simulink model "CAN_basics"  (R2019a)
settings: Solver=FixedStepAuto  StartTime=0.0  StopTime=inf  RelTol=1e-3
InitFcn:
  | InitFcn
undefined symbols (not defined in the file or in its folder): CAN_ID_Frequencydata, CAN_ID_RAW_A0, CAN_ID_RAW_A1, CAN_ID_RAW_B0, CAN_ID_RAW_B1, CAN_ID_RAW_C0, CAN_ID_RAW_C1, CAN_ID_RAW_D0, CAN_ID_RAW_D1, CAN_ID_Timedata, canChannel
libraries: etargetslib x26, canmsglib x18, canlib x9, simulink x2
settings Model: Creator=abl  LastModifiedBy=abl

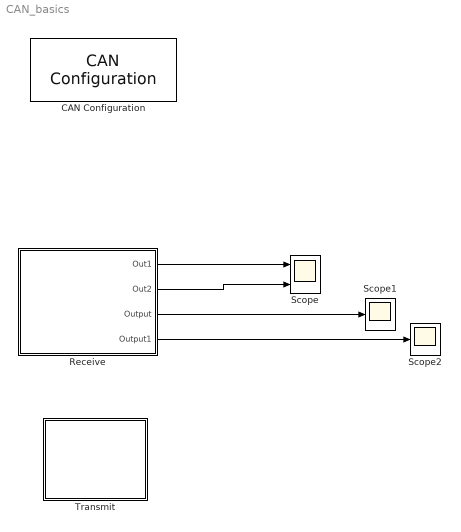
== system CAN_basics ==
  CAN Configuration : canlib/CAN Configuration  BlockHandle=2.0001  DeviceMenu=Vector VN1610 1 (Channel 1)  Device=Vector VN1610 1 (Channel 1)  ObjConstructor=canChannel('Vector', 'VN1610 1', 1)  BusSpeed=500000  EnableBitParameters=off  SJW=1  TSEG1=4  TSEG2=3  NSamples=1  AckMode=Normal
      settings: SourceProductName=Vehicle Network Toolbox  SourceProductBaseCode=VN
  Receive : Subsystem
  Scope : Scope  NumInputPorts=2
  Scope1 : Scope
  Scope2 : Scope
  Transmit : Subsystem
  wires:
  Receive/1(Out1) -> Scope/1
  Receive/2(Out2) -> Scope/2
  Receive/3(Output) -> Scope1/1
  Receive/4(Output1) -> Scope2/1

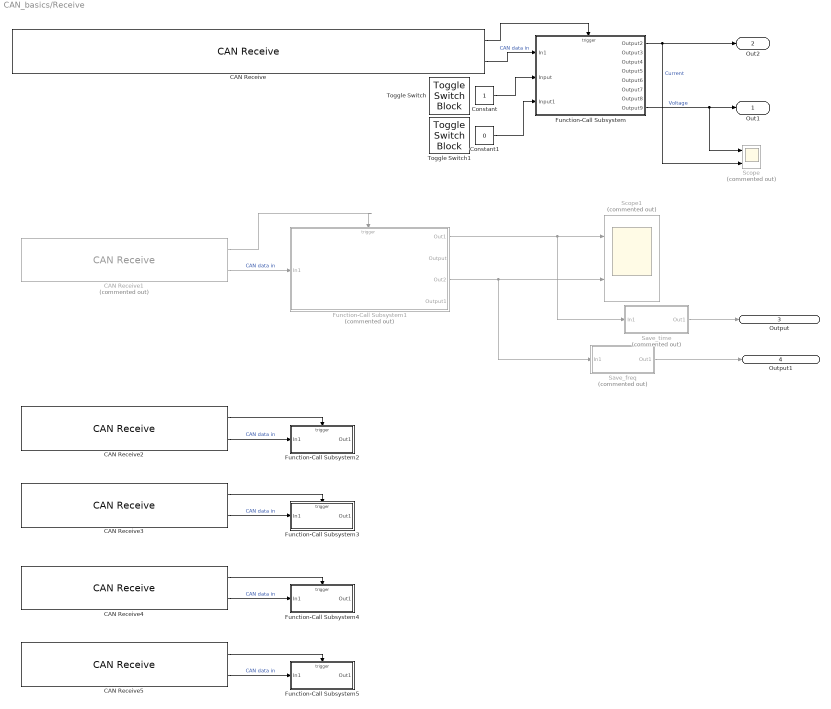
== system CAN_basics/Receive ==
  CAN Receive : canlib/CAN Receive  BlockHandle=4.0001  DeviceMenu=Vector VN1610 1 (Channel 1)  Device=Vector VN1610 1 (Channel 1)  ObjConstructor=canChannel('Vector', 'VN1610 1', 1)  EnableStandardIDsFilter=off  StandardIDs=[CAN_ID_RAW_A0;CAN_ID_RAW_A1;CAN_ID_RAW_B0;CAN_ID_RAW_B1;CAN_ID_RAW_C0;CAN_ID_RAW_C1;CAN_ID_RAW_D0;CAN_ID_RAW_D1]  EnableExtendedIDsFilter=off  ExtendedIDs=0  SampleTime=-1  MsgsPerTimestep=all  StdIDsCombo=Allow only  ExtIDsCombo=Block all  InternalFilterUpdateStatus=on  BusOutput=off
      settings: SourceProductName=Vehicle Network Toolbox  SourceProductBaseCode=VN
  CAN Receive1 : canlib/CAN Receive  Commented=on  BlockHandle=5.0001  DeviceMenu=Vector VN1610 1 (Channel 1)  Device=Vector VN1610 1 (Channel 1)  ObjConstructor=canChannel('Vector', 'VN1610 1', 1)  EnableStandardIDsFilter=off  StandardIDs=[CAN_ID_Timedata;CAN_ID_Frequencydata]  EnableExtendedIDsFilter=off  ExtendedIDs=0  SampleTime=-1  MsgsPerTimestep=all  StdIDsCombo=Allow only  ExtIDsCombo=Block all  InternalFilterUpdateStatus=on  BusOutput=off
      settings: SourceProductName=Vehicle Network Toolbox  SourceProductBaseCode=VN
  CAN Receive2 : canlib/CAN Receive  BlockHandle=6.0001  DeviceMenu=Vector VN1610 1 (Channel 1)  Device=Vector VN1610 1 (Channel 1)  ObjConstructor=canChannel('Vector', 'VN1610 1', 1)  EnableStandardIDsFilter=off  StandardIDs=CAN_ID_Timedata  EnableExtendedIDsFilter=off  ExtendedIDs=0  SampleTime=-1  MsgsPerTimestep=all  StdIDsCombo=Allow only  ExtIDsCombo=Block all  InternalFilterUpdateStatus=on  BusOutput=off
      settings: SourceProductName=Vehicle Network Toolbox  SourceProductBaseCode=VN
  CAN Receive3 : canlib/CAN Receive  BlockHandle=7.0001  DeviceMenu=Vector VN1610 1 (Channel 1)  Device=Vector VN1610 1 (Channel 1)  ObjConstructor=canChannel('Vector', 'VN1610 1', 1)  EnableStandardIDsFilter=off  StandardIDs=CAN_ID_Frequencydata  EnableExtendedIDsFilter=off  ExtendedIDs=0  SampleTime=-1  MsgsPerTimestep=all  StdIDsCombo=Allow only  ExtIDsCombo=Block all  InternalFilterUpdateStatus=on  BusOutput=off
      settings: SourceProductName=Vehicle Network Toolbox  SourceProductBaseCode=VN
  CAN Receive4 : canlib/CAN Receive  BlockHandle=1226.0002  DeviceMenu=Vector VN1610 1 (Channel 1)  Device=Vector VN1610 1 (Channel 1)  ObjConstructor=canChannel('Vector', 'VN1610 1', 1)  EnableStandardIDsFilter=off  StandardIDs=CAN_ID_Timedata_float  EnableExtendedIDsFilter=off  ExtendedIDs=0  SampleTime=-1  MsgsPerTimestep=1  StdIDsCombo=Allow only  ExtIDsCombo=Block all  InternalFilterUpdateStatus=on  BusOutput=off
      settings: SourceProductName=Vehicle Network Toolbox  SourceProductBaseCode=VN
  CAN Receive5 : canlib/CAN Receive  BlockHandle=1227.0002  DeviceMenu=Vector VN1610 1 (Channel 1)  Device=Vector VN1610 1 (Channel 1)  ObjConstructor=canChannel('Vector', 'VN1610 1', 1)  EnableStandardIDsFilter=off  StandardIDs=CAN_ID_Frequencydata_float  EnableExtendedIDsFilter=off  ExtendedIDs=0  SampleTime=-1  MsgsPerTimestep=1  StdIDsCombo=Allow only  ExtIDsCombo=Block all  InternalFilterUpdateStatus=on  BusOutput=off
      settings: SourceProductName=Vehicle Network Toolbox  SourceProductBaseCode=VN
  Constant : Constant
  Constant1 : Constant  Value=0
  Function-Call Subsystem : Subsystem  TreatAsAtomicUnit=on
  Function-Call Subsystem1 : Subsystem  Commented=on  TreatAsAtomicUnit=on
  Function-Call Subsystem2 : Subsystem  TreatAsAtomicUnit=on
  Function-Call Subsystem3 : Subsystem  TreatAsAtomicUnit=on
  Function-Call Subsystem4 : Subsystem  TreatAsAtomicUnit=on
  Function-Call Subsystem5 : Subsystem  TreatAsAtomicUnit=on
  Save_freq : Subsystem  Commented=on
  Save_time : Subsystem  Commented=on
  Scope : Scope  Commented=on  NumInputPorts=2
  Scope1 : Scope  Commented=on  NumInputPorts=2
  Toggle Switch : ToggleSwitchBlock  LabelPosition=Hide
      settings: Values={{'double', 'int16'}, [1 0]}
  Toggle Switch1 : ToggleSwitchBlock  LabelPosition=Hide
      settings: Values={{'8 CAN messages', '2 CAN messages'}, [1 0]}
  Out1 : Outport
  Out2 : Outport  Port=2
  Output : Outport  Port=3
  Output1 : Outport  Port=4
  wires:
  Function-Call Subsystem/8(Output9) -> Scope/1, Out1/1  "Voltage"
  Constant/1 -> Function-Call Subsystem/2(Input)
  CAN Receive/2 -> Function-Call Subsystem/1(In1)  "CAN data in"
  Constant1/1 -> Function-Call Subsystem/3(Input1)
  CAN Receive/1 -> Function-Call Subsystem/Trigger
  Function-Call Subsystem/1(Output2) -> Scope/2, Out2/1  "Current"
  CAN Receive1/1 -> Function-Call Subsystem1/Trigger
  CAN Receive1/2 -> Function-Call Subsystem1/1(In1)  "CAN data in"
  Function-Call Subsystem1/1(Out1) -> Save_time/1(In1), Scope1/1
  Function-Call Subsystem1/3(Out2) -> Save_freq/1(In1), Scope1/2
  Save_time/1(Out1) -> Output/1
  Save_freq/1(Out1) -> Output1/1
  CAN Receive2/2 -> Function-Call Subsystem2/1(In1)  "CAN data in"
  CAN Receive2/1 -> Function-Call Subsystem2/Trigger
  CAN Receive3/1 -> Function-Call Subsystem3/Trigger
  CAN Receive3/2 -> Function-Call Subsystem3/1(In1)  "CAN data in"
  CAN Receive4/1 -> Function-Call Subsystem4/Trigger
  CAN Receive4/2 -> Function-Call Subsystem4/1(In1)  "CAN data in"
  CAN Receive5/2 -> Function-Call Subsystem5/1(In1)  "CAN data in"
  CAN Receive5/1 -> Function-Call Subsystem5/Trigger

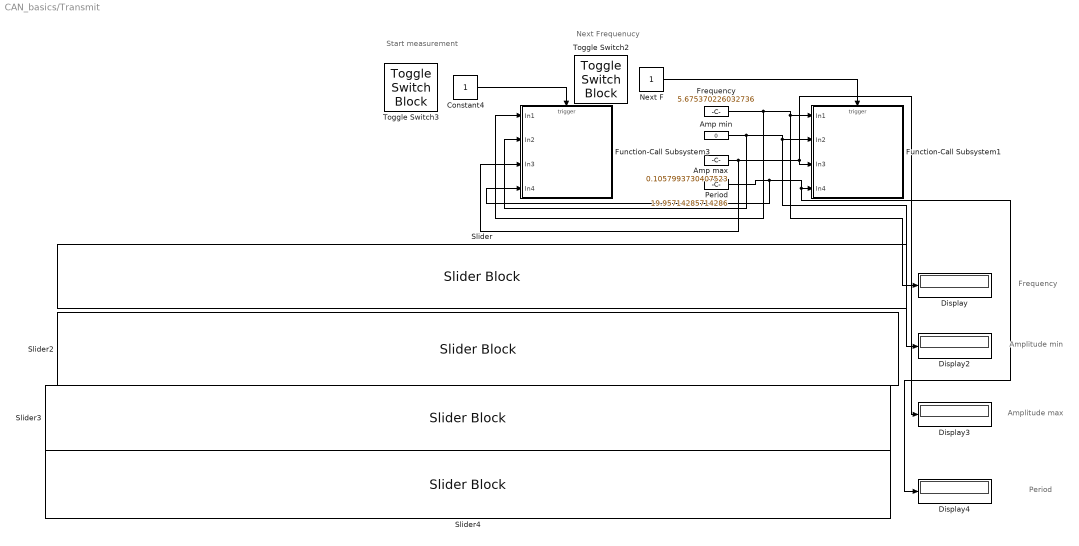
== system CAN_basics/Transmit ==
  note: Amplitude min
  note: Frequency
  note: Next Frequenucy
  note: Start measurement
  note: Amplitude max
  note: Period
  Amp max : Constant  Value=0.1057993730407523
  Amp min : Constant  Value=0
  Constant4 : Constant
  Display{,2..4} (4 alike) : Display
  Frequency : Constant  Value=5.675370226032736  OutDataTypeStr=uint16
  Function-Call Subsystem1 : Subsystem  TreatAsAtomicUnit=on
  Function-Call Subsystem3 : Subsystem  TreatAsAtomicUnit=on
  Next F : Constant
  Period : Constant  Value=19.95714285714286  OutDataTypeStr=uint16
  Slider : SliderBlock  ScaleMin=1  ScaleMax=4000
  Slider2 : SliderBlock  ScaleMax=5
  Slider3 : SliderBlock  ScaleMax=5
  Slider4 : SliderBlock  ScaleMin=1  ScaleMax=30  TickInterval=1
  Toggle Switch2 : ToggleSwitchBlock  LabelPosition=Hide
      settings: Values={{'Send message', 'Send message'}, [1 0]}
  Toggle Switch3 : ToggleSwitchBlock  LabelPosition=Hide
      settings: Values={{'Send message', 'Send message'}, [1 0]}
  wires:
  Amp min/1 -> Function-Call Subsystem3/2(In2), Display2/1, Function-Call Subsystem1/2(In2)
  Amp max/1 -> Display3/1, Function-Call Subsystem1/3(In3), Function-Call Subsystem3/3(In3)
  Period/1 -> Function-Call Subsystem3/4(In4), Display4/1, Function-Call Subsystem1/4(In4)
  Constant4/1 -> Function-Call Subsystem3/Trigger
  Next F/1 -> Function-Call Subsystem1/Trigger
  Frequency/1 -> Function-Call Subsystem3/1(In1), Display/1, Function-Call Subsystem1/1(In1)

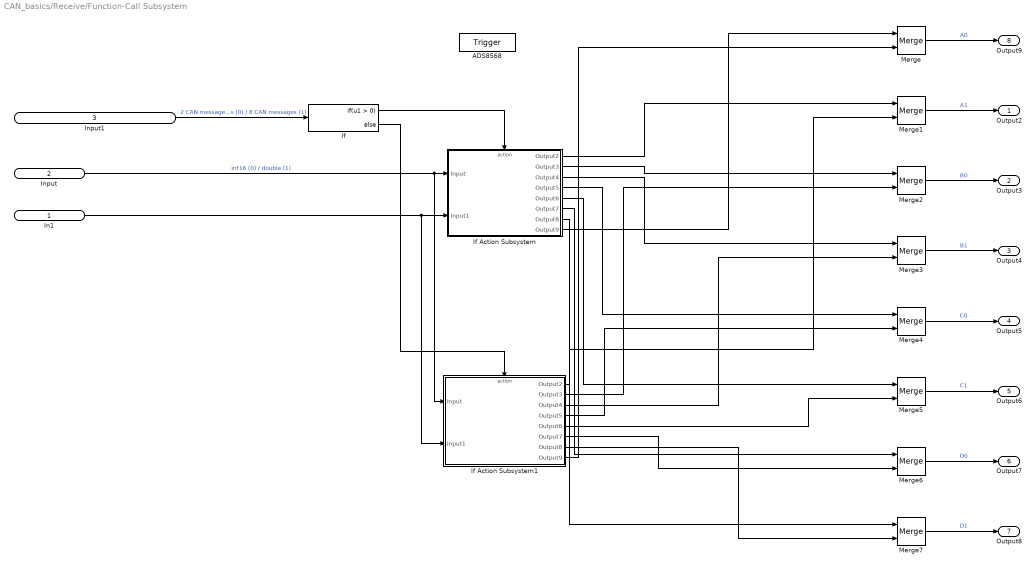
== system CAN_basics/Receive/Function-Call Subsystem ==
  In1 : Inport  Description=CAN data in
  Input : Inport  Port=2
  Input1 : Inport  Port=3
  ADS8568 : TriggerPort  TriggerType=function-call  VariantControl=Variant
  If : If
  If Action Subsystem : Subsystem  TreatAsAtomicUnit=on
  If Action Subsystem1 : Subsystem  TreatAsAtomicUnit=on
  Merge{,1..7} (8 alike) : Merge
  Output2 : Outport
  Output3 : Outport  Port=2
  Output4 : Outport  Port=3
  Output5 : Outport  Port=4
  Output6 : Outport  Port=5
  Output7 : Outport  Port=6
  Output8 : Outport  Port=7
  Output9 : Outport  Port=8
  wires:
  Input/1 -> If Action Subsystem1/1(Input), If Action Subsystem/1(Input)  "int16 (0) / double (1)"
  In1/1 -> If Action Subsystem1/2(Input1), If Action Subsystem/2(Input1)
  If/1 -> If Action Subsystem/Action
  Input1/1 -> If/1  "2 CAN messages (0) / 8 CAN messages (1)"
  If Action Subsystem/8(Output9) -> Merge/1
  If/2 -> If Action Subsystem1/Action
  Merge7/1 -> Output8/1  "D1"
  Merge6/1 -> Output7/1  "D0"
  Merge5/1 -> Output6/1  "C1"
  Merge4/1 -> Output5/1  "C0"
  Merge3/1 -> Output4/1  "B1"
  Merge2/1 -> Output3/1  "B0"
  Merge1/1 -> Output2/1  "A1"
  Merge/1 -> Output9/1  "A0"
  If Action Subsystem/1(Output2) -> Merge1/1
  If Action Subsystem/2(Output3) -> Merge2/1
  If Action Subsystem/3(Output4) -> Merge3/1
  If Action Subsystem/4(Output5) -> Merge4/1
  If Action Subsystem/5(Output6) -> Merge5/1
  If Action Subsystem/6(Output7) -> Merge6/1
  If Action Subsystem/7(Output8) -> Merge7/1
  If Action Subsystem1/8(Output9) -> Merge/2
  If Action Subsystem1/1(Output2) -> Merge1/2
  If Action Subsystem1/2(Output3) -> Merge2/2
  If Action Subsystem1/3(Output4) -> Merge3/2
  If Action Subsystem1/7(Output8) -> Merge7/2
  If Action Subsystem1/6(Output7) -> Merge6/2
  If Action Subsystem1/5(Output6) -> Merge5/2
  If Action Subsystem1/4(Output5) -> Merge4/2

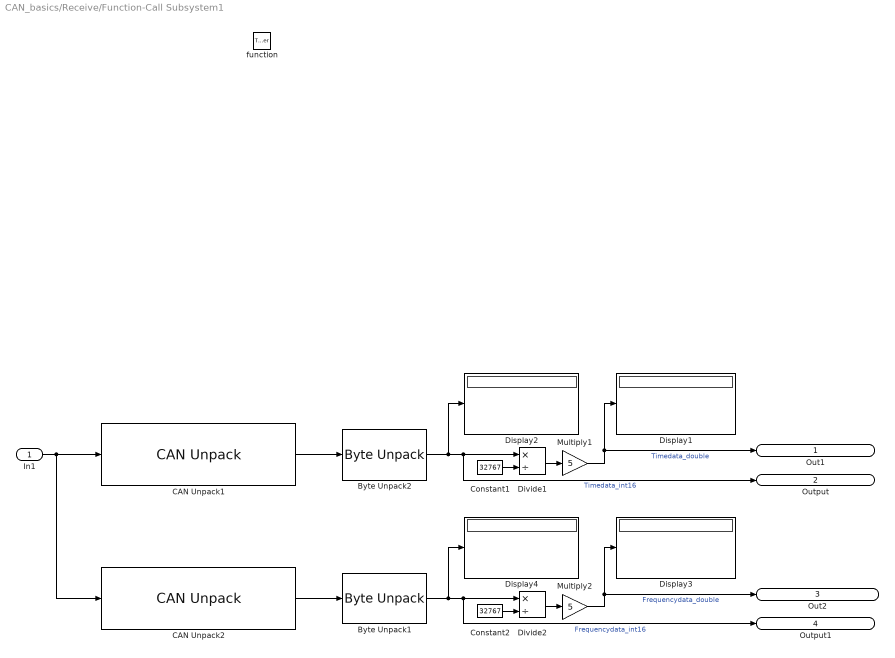
== system CAN_basics/Receive/Function-Call Subsystem1 ==
  In1 : Inport
  function : TriggerPort  TriggerType=function-call  VariantControl=Variant
  Byte Unpack1 : etargetslib/Byte Unpack  dimensions={[4]}  datatypes={'uint16'}  byteAlign=1
      settings: SourceProductName=MATLAB Coder
  Byte Unpack2 : etargetslib/Byte Unpack  dimensions={[4]}  datatypes={'uint16'}  byteAlign=1
      settings: SourceProductName=MATLAB Coder
  CAN Unpack1 : canmsglib/CAN Unpack  MsgList=(none)  MsgName=Timedata  MsgIDType=Standard (11-bit identifier)  MsgIdentifier=CAN_ID_Timedata  MsgLength=8  SignalInfo=A0$0$16$1$1$1$0$1$0$-Inf$Inf$#  NSignals=1  IDPort=off  TimestampPort=off  ErrorPort=off  RemotePort=off  LengthPort=off  StatusPort=off  StartBits=str2num('[int32(0)]')  SignalSizes=str2num('[int32(16)]')  ByteOrders=str2num('[int32(1)]')  DataTypes=str2num('[int32(1)]')  MultiplexTypes=str2num('[int32(1)]')  MultiplexValues=str2num('[double(0)]')  Factors=str2num('[double(1)]')  Offsets=str2num('[double(0)]')  Minimums=str2num('[double(-Inf)]')  Maximums=str2num('[double(Inf)]')  ApplyMinMax=off
      settings: SourceProductName=Vehicle Network Toolbox  SourceProductBaseCode=VN  DataFormat=raw data
  CAN Unpack2 : canmsglib/CAN Unpack  MsgList=(none)  MsgName=Frequencydata  MsgIDType=Standard (11-bit identifier)  MsgIdentifier=CAN_ID_Frequencydata  MsgLength=8  SignalInfo=A0$0$16$1$1$1$0$1$0$-Inf$Inf$#  NSignals=1  IDPort=off  TimestampPort=off  ErrorPort=off  RemotePort=off  LengthPort=off  StatusPort=off  StartBits=str2num('[int32(0)]')  SignalSizes=str2num('[int32(16)]')  ByteOrders=str2num('[int32(1)]')  DataTypes=str2num('[int32(1)]')  MultiplexTypes=str2num('[int32(1)]')  MultiplexValues=str2num('[double(0)]')  Factors=str2num('[double(1)]')  Offsets=str2num('[double(0)]')  Minimums=str2num('[double(-Inf)]')  Maximums=str2num('[double(Inf)]')  ApplyMinMax=off
      settings: SourceProductName=Vehicle Network Toolbox  SourceProductBaseCode=VN  DataFormat=raw data
  Constant1 : Constant  Value=32767
  Constant2 : Constant  Value=32767
  Display{1..4} (4 alike) : Display
      settings: Format=decimal (Stored Integer)
  Divide1 : Product  Inputs=*/
  Divide2 : Product  Inputs=*/
  Multiply1 : Gain  Gain=5
  Multiply2 : Gain  Gain=5
  Out1 : Outport
  Output : Outport  Port=2
  Out2 : Outport  Port=3
  Output1 : Outport  Port=4
  wires:
  CAN Unpack1/1 -> Byte Unpack2/1
  Divide1/1 -> Multiply1/1
  Multiply1/1 -> Out1/1, Display1/1  "Timedata_double"
  Constant1/1 -> Divide1/2
  Byte Unpack2/1 -> Output/1, Divide1/1, Display2/1  "Timedata_int16"
  Byte Unpack1/1 -> Output1/1, Divide2/1, Display4/1  "Frequencydata_int16"
  Constant2/1 -> Divide2/2
  Divide2/1 -> Multiply2/1
  Multiply2/1 -> Out2/1, Display3/1  "Frequencydata_double"
  CAN Unpack2/1 -> Byte Unpack1/1
  In1/1 -> CAN Unpack2/1, CAN Unpack1/1

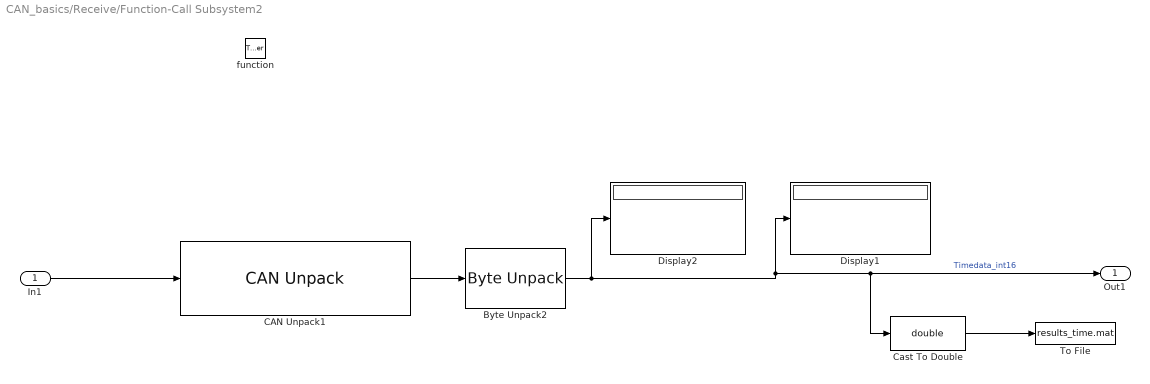
== system CAN_basics/Receive/Function-Call Subsystem2 ==
  In1 : Inport
  function : TriggerPort  TriggerType=function-call  VariantControl=Variant
  Byte Unpack2 : etargetslib/Byte Unpack  dimensions={[4]}  datatypes={'int16'}  byteAlign=1
      settings: SourceProductName=MATLAB Coder
  CAN Unpack1 : canmsglib/CAN Unpack  MsgList=(none)  MsgName=Timedata  MsgIDType=Standard (11-bit identifier)  MsgIdentifier=CAN_ID_Timedata  MsgLength=8  SignalInfo=A0$0$16$1$1$1$0$1$0$-Inf$Inf$#  NSignals=1  IDPort=off  TimestampPort=off  ErrorPort=off  RemotePort=off  LengthPort=off  StatusPort=off  StartBits=str2num('[int32(0)]')  SignalSizes=str2num('[int32(16)]')  ByteOrders=str2num('[int32(1)]')  DataTypes=str2num('[int32(1)]')  MultiplexTypes=str2num('[int32(1)]')  MultiplexValues=str2num('[double(0)]')  Factors=str2num('[double(1)]')  Offsets=str2num('[double(0)]')  Minimums=str2num('[double(-Inf)]')  Maximums=str2num('[double(Inf)]')  ApplyMinMax=off
      settings: SourceProductName=Vehicle Network Toolbox  SourceProductBaseCode=VN  DataFormat=raw data
  Cast To Double : DataTypeConversion  OutDataTypeStr=double
  Display1 : Display
      settings: Format=decimal (Stored Integer)
  Display2 : Display
      settings: Format=decimal (Stored Integer)
  To File : ToFile  Filename=results_time.mat  MatrixName=results_time
  Out1 : Outport
  wires:
  Byte Unpack2/1 -> Cast To Double/1, Out1/1, Display1/1, Display2/1  "Timedata_int16"
  CAN Unpack1/1 -> Byte Unpack2/1
  In1/1 -> CAN Unpack1/1
  Cast To Double/1 -> To File/1

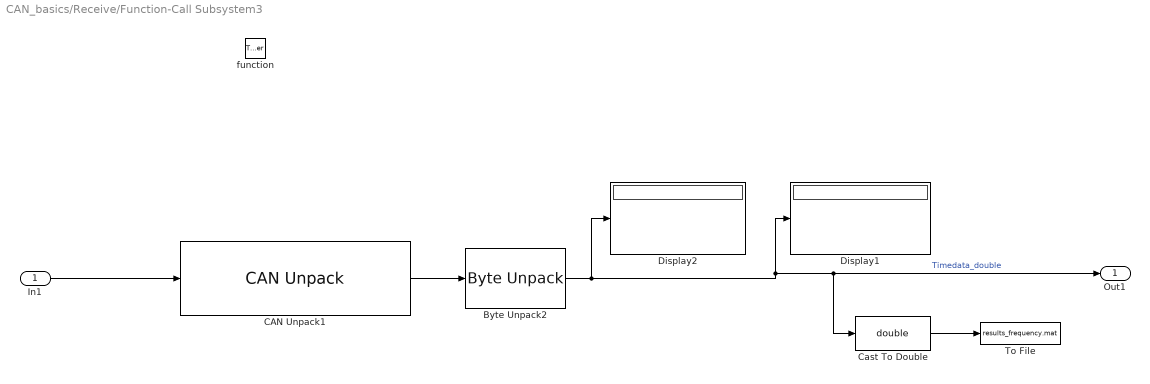
== system CAN_basics/Receive/Function-Call Subsystem3 ==
  In1 : Inport
  function : TriggerPort  TriggerType=function-call  VariantControl=Variant
  Byte Unpack2 : etargetslib/Byte Unpack  dimensions={[4]}  datatypes={'int16'}  byteAlign=1
      settings: SourceProductName=MATLAB Coder
  CAN Unpack1 : canmsglib/CAN Unpack  MsgList=(none)  MsgName=Frequencydata  MsgIDType=Standard (11-bit identifier)  MsgIdentifier=CAN_ID_Frequencydata  MsgLength=8  SignalInfo=A0$0$16$1$1$1$0$1$0$-Inf$Inf$#  NSignals=1  IDPort=off  TimestampPort=off  ErrorPort=off  RemotePort=off  LengthPort=off  StatusPort=off  StartBits=str2num('[int32(0)]')  SignalSizes=str2num('[int32(16)]')  ByteOrders=str2num('[int32(1)]')  DataTypes=str2num('[int32(1)]')  MultiplexTypes=str2num('[int32(1)]')  MultiplexValues=str2num('[double(0)]')  Factors=str2num('[double(1)]')  Offsets=str2num('[double(0)]')  Minimums=str2num('[double(-Inf)]')  Maximums=str2num('[double(Inf)]')  ApplyMinMax=off
      settings: SourceProductName=Vehicle Network Toolbox  SourceProductBaseCode=VN  DataFormat=raw data
  Cast To Double : DataTypeConversion  OutDataTypeStr=double
  Display1 : Display
      settings: Format=decimal (Stored Integer)
  Display2 : Display
      settings: Format=decimal (Stored Integer)
  To File : ToFile  Filename=results_frequency.mat  MatrixName=results_frequency
  Out1 : Outport
  wires:
  Byte Unpack2/1 -> Cast To Double/1, Out1/1, Display1/1, Display2/1  "Timedata_double"
  CAN Unpack1/1 -> Byte Unpack2/1
  In1/1 -> CAN Unpack1/1
  Cast To Double/1 -> To File/1

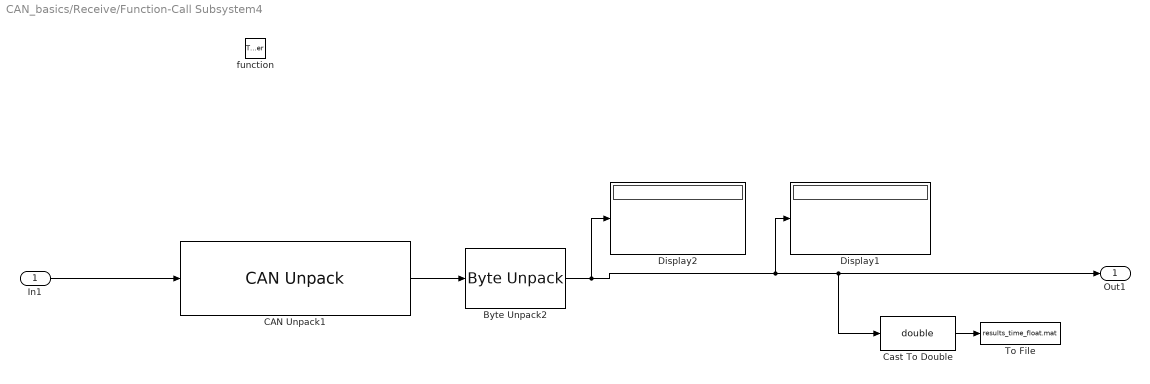
== system CAN_basics/Receive/Function-Call Subsystem4 ==
  In1 : Inport
  function : TriggerPort  TriggerType=function-call  VariantControl=Variant
  Byte Unpack2 : etargetslib/Byte Unpack  dimensions={[2]}  datatypes={'single'}  byteAlign=1
      settings: SourceProductName=MATLAB Coder
  CAN Unpack1 : canmsglib/CAN Unpack  MsgList=(none)  MsgName=Timedata  MsgIDType=Standard (11-bit identifier)  MsgIdentifier=CAN_ID_Timedata_float  MsgLength=8  SignalInfo=A0$0$16$1$1$1$0$1$0$-Inf$Inf$#  NSignals=1  IDPort=off  TimestampPort=off  ErrorPort=off  RemotePort=off  LengthPort=off  StatusPort=off  StartBits=str2num('[int32(0)]')  SignalSizes=str2num('[int32(16)]')  ByteOrders=str2num('[int32(1)]')  DataTypes=str2num('[int32(1)]')  MultiplexTypes=str2num('[int32(1)]')  MultiplexValues=str2num('[double(0)]')  Factors=str2num('[double(1)]')  Offsets=str2num('[double(0)]')  Minimums=str2num('[double(-Inf)]')  Maximums=str2num('[double(Inf)]')  ApplyMinMax=off
      settings: SourceProductName=Vehicle Network Toolbox  SourceProductBaseCode=VN  DataFormat=raw data
  Cast To Double : DataTypeConversion  OutDataTypeStr=double
  Display1 : Display
      settings: Format=decimal (Stored Integer)
  Display2 : Display
      settings: Format=decimal (Stored Integer)
  To File : ToFile  Filename=results_time_float.mat  MatrixName=results_time_float
  Out1 : Outport
  wires:
  Byte Unpack2/1 -> Cast To Double/1, Out1/1, Display1/1, Display2/1
  CAN Unpack1/1 -> Byte Unpack2/1
  In1/1 -> CAN Unpack1/1
  Cast To Double/1 -> To File/1

== system CAN_basics/Receive/Function-Call Subsystem5 ==
  In1 : Inport
  function : TriggerPort  TriggerType=function-call  VariantControl=Variant
  Byte Unpack2 : etargetslib/Byte Unpack  dimensions={[2]}  datatypes={'single'}  byteAlign=1
      settings: SourceProductName=MATLAB Coder
  CAN Unpack1 : canmsglib/CAN Unpack  MsgList=(none)  MsgName=Frequencydata  MsgIDType=Standard (11-bit identifier)  MsgIdentifier=CAN_ID_Frequencydata_float  MsgLength=8  SignalInfo=A0$0$16$1$1$1$0$1$0$-Inf$Inf$#  NSignals=1  IDPort=off  TimestampPort=off  ErrorPort=off  RemotePort=off  LengthPort=off  StatusPort=off  StartBits=str2num('[int32(0)]')  SignalSizes=str2num('[int32(16)]')  ByteOrders=str2num('[int32(1)]')  DataTypes=str2num('[int32(1)]')  MultiplexTypes=str2num('[int32(1)]')  MultiplexValues=str2num('[double(0)]')  Factors=str2num('[double(1)]')  Offsets=str2num('[double(0)]')  Minimums=str2num('[double(-Inf)]')  Maximums=str2num('[double(Inf)]')  ApplyMinMax=off
      settings: SourceProductName=Vehicle Network Toolbox  SourceProductBaseCode=VN  DataFormat=raw data
  Cast To Double : DataTypeConversion  OutDataTypeStr=double
  Display1 : Display
      settings: Format=decimal (Stored Integer)
  Display2 : Display
      settings: Format=decimal (Stored Integer)
  To File : ToFile  Filename=results_frequency_float.mat  MatrixName=results_frequency_float
  Out1 : Outport
  wires:
  Byte Unpack2/1 -> Display1/1, Out1/1, Cast To Double/1, Display2/1
  CAN Unpack1/1 -> Byte Unpack2/1
  In1/1 -> CAN Unpack1/1
  Cast To Double/1 -> To File/1

== system CAN_basics/Receive/Save_freq ==
  In1 : Inport
  Detect Change : simulink/Logic and Bit Operations/Detect Change  vinit=0  OutDataTypeStr=boolean
  Triggered Subsystem : Subsystem  TreatAsAtomicUnit=on
  Out1 : Outport
  wires:
  In1/1 -> Triggered Subsystem/1(In1), Detect Change/1
  Detect Change/1 -> Triggered Subsystem/Trigger
  Triggered Subsystem/1(Out1) -> Out1/1

== system CAN_basics/Receive/Save_time ==
  In1 : Inport
  Detect Change : simulink/Logic and Bit Operations/Detect Change  vinit=0  OutDataTypeStr=boolean
  Triggered Subsystem : Subsystem  TreatAsAtomicUnit=on
  Out1 : Outport
  wires:
  In1/1 -> Triggered Subsystem/1(In1), Detect Change/1
  Detect Change/1 -> Triggered Subsystem/Trigger
  Triggered Subsystem/1(Out1) -> Out1/1

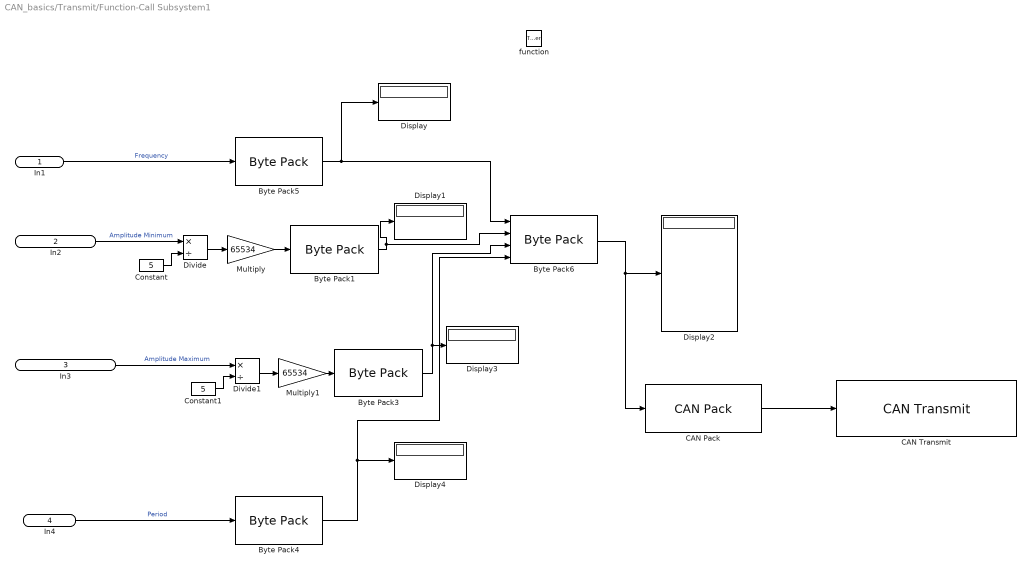
== system CAN_basics/Transmit/Function-Call Subsystem1 ==
  In1 : Inport
  In2 : Inport  Port=2
  In3 : Inport  Port=3
  In4 : Inport  Port=4
  function : TriggerPort  TriggerType=either  VariantControl=Variant
  Byte Pack{1,3..5} (4 alike) : etargetslib/Byte Pack  datatypes={'uint16'}  byteAlign=1
      settings: SourceProductName=MATLAB Coder
  Byte Pack6 : etargetslib/Byte Pack  datatypes={'uint8','uint8','uint8','uint8'}  byteAlign=1
      settings: SourceProductName=MATLAB Coder
  CAN Pack : canmsglib/CAN Pack  MsgList=(none)  MsgName=CAN Msg  MsgIDType=Standard (11-bit identifier)  MsgIdentifier=CAN_ID_Next_F  MsgLength=8  NSignals=0  StartBits=0  SignalSizes=0  ByteOrders=0  DataTypes=0  MultiplexTypes=0  MultiplexValues=0  Factors=0  Offsets=0  Minimums=0  Maximums=0  Remote=off  ApplyMinMax=off  BusOutput=off
      settings: SourceProductName=Vehicle Network Toolbox  SourceProductBaseCode=VN  DataFormat=raw data
  CAN Transmit : canlib/CAN Transmit  BlockHandle=541.0004  DeviceMenu=Vector VN1610 1 (Channel 1)  Device=Vector VN1610 1 (Channel 1)  ObjConstructor=canChannel('Vector', 'VN1610 1', 1)  EnablePeriodicTransmit=off  MessagePeriod=1.000
      settings: SourceProductName=Vehicle Network Toolbox  SourceProductBaseCode=VN
  Constant : Constant  Value=5
  Constant1 : Constant  Value=5
  Display{,1..4} (5 alike) : Display
  Divide : Product  Inputs=*/
  Divide1 : Product  Inputs=*/
  Multiply : Gain  Gain=65534  OutDataTypeStr=uint16
  Multiply1 : Gain  Gain=65534  OutDataTypeStr=uint16
  wires:
  CAN Pack/1 -> CAN Transmit/1
  In1/1 -> Byte Pack5/1  "Frequency"
  Byte Pack5/1 -> Byte Pack6/1, Display/1
  In2/1 -> Divide/1  "Amplitude Minimum"
  Constant/1 -> Divide/2
  Divide/1 -> Multiply/1
  Multiply/1 -> Byte Pack1/1
  Byte Pack1/1 -> Display1/1, Byte Pack6/2
  Byte Pack6/1 -> CAN Pack/1, Display2/1
  Divide1/1 -> Multiply1/1
  Constant1/1 -> Divide1/2
  In3/1 -> Divide1/1  "Amplitude Maximum"
  Multiply1/1 -> Byte Pack3/1
  Byte Pack3/1 -> Byte Pack6/3, Display3/1
  In4/1 -> Byte Pack4/1  "Period"
  Byte Pack4/1 -> Byte Pack6/4, Display4/1

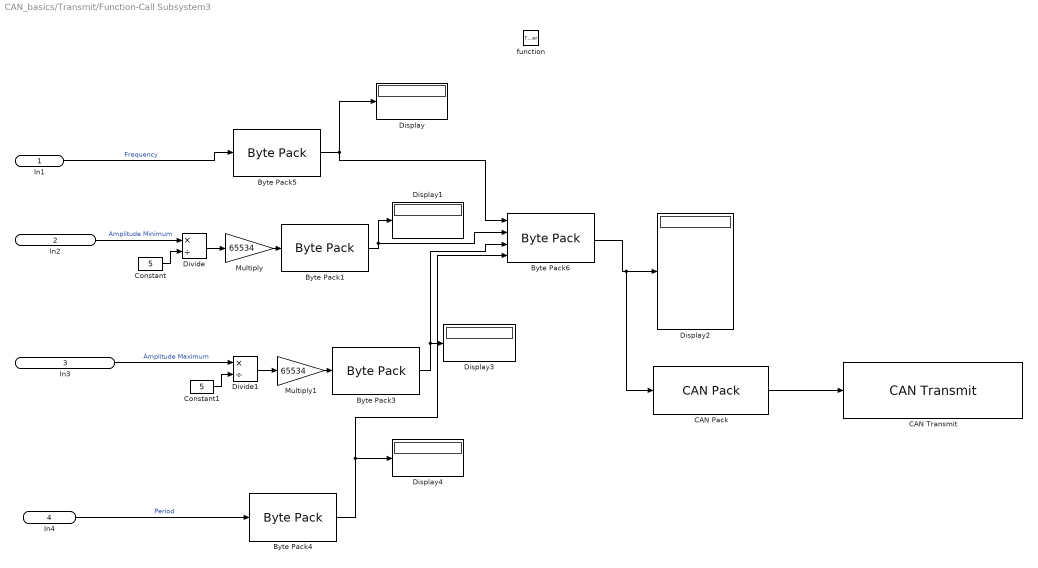
== system CAN_basics/Transmit/Function-Call Subsystem3 ==
  In1 : Inport
  In2 : Inport  Port=2
  In3 : Inport  Port=3
  In4 : Inport  Port=4
  function : TriggerPort  TriggerType=either  VariantControl=Variant
  Byte Pack{1,3..5} (4 alike) : etargetslib/Byte Pack  datatypes={'uint16'}  byteAlign=1
      settings: SourceProductName=MATLAB Coder
  Byte Pack6 : etargetslib/Byte Pack  datatypes={'uint8','uint8','uint8','uint8'}  byteAlign=2
      settings: SourceProductName=MATLAB Coder
  CAN Pack : canmsglib/CAN Pack  MsgList=(none)  MsgName=CAN Msg  MsgIDType=Standard (11-bit identifier)  MsgIdentifier=CAN_ID_Start_M  MsgLength=8  NSignals=0  StartBits=0  SignalSizes=0  ByteOrders=0  DataTypes=0  MultiplexTypes=0  MultiplexValues=0  Factors=0  Offsets=0  Minimums=0  Maximums=0  Remote=off  ApplyMinMax=off  BusOutput=off
      settings: SourceProductName=Vehicle Network Toolbox  SourceProductBaseCode=VN  DataFormat=raw data
  CAN Transmit : canlib/CAN Transmit  BlockHandle=591.0004  DeviceMenu=Vector VN1610 1 (Channel 1)  Device=Vector VN1610 1 (Channel 1)  ObjConstructor=canChannel('Vector', 'VN1610 1', 1)  EnablePeriodicTransmit=off  MessagePeriod=1.000
      settings: SourceProductName=Vehicle Network Toolbox  SourceProductBaseCode=VN
  Constant : Constant  Value=5
  Constant1 : Constant  Value=5
  Display{,1..4} (5 alike) : Display
  Divide : Product  Inputs=*/
  Divide1 : Product  Inputs=*/
  Multiply : Gain  Gain=65534  OutDataTypeStr=uint16
  Multiply1 : Gain  Gain=65534  OutDataTypeStr=uint16
  wires:
  CAN Pack/1 -> CAN Transmit/1
  In1/1 -> Byte Pack5/1  "Frequency"
  Byte Pack5/1 -> Byte Pack6/1, Display/1
  In2/1 -> Divide/1  "Amplitude Minimum"
  Constant/1 -> Divide/2
  Divide/1 -> Multiply/1
  Multiply/1 -> Byte Pack1/1
  Byte Pack1/1 -> Display1/1, Byte Pack6/2
  Byte Pack6/1 -> CAN Pack/1, Display2/1
  Divide1/1 -> Multiply1/1
  Constant1/1 -> Divide1/2
  In3/1 -> Divide1/1  "Amplitude Maximum"
  Multiply1/1 -> Byte Pack3/1
  Byte Pack3/1 -> Byte Pack6/3, Display3/1
  In4/1 -> Byte Pack4/1  "Period"
  Byte Pack4/1 -> Byte Pack6/4, Display4/1

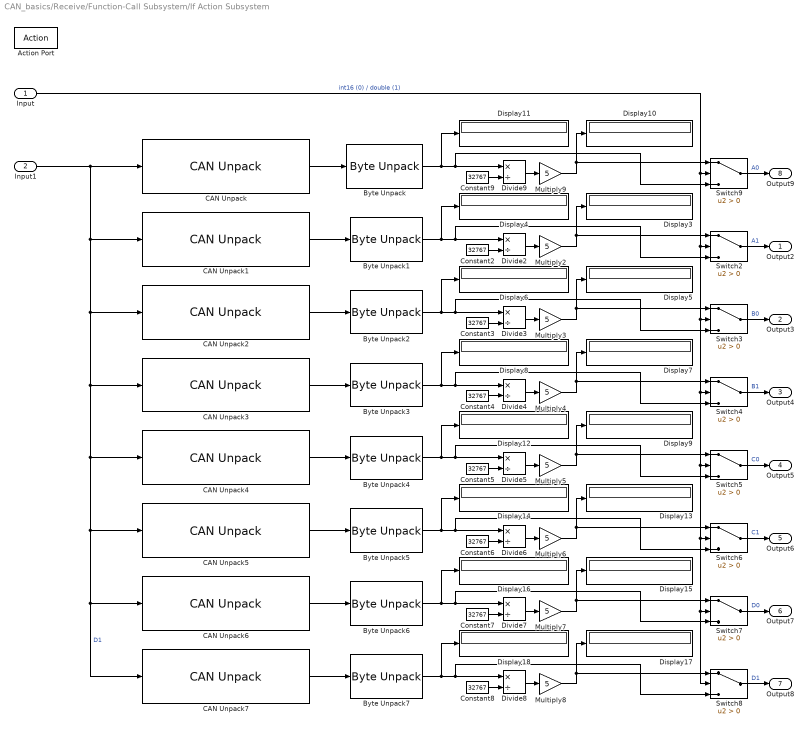
== system CAN_basics/Receive/Function-Call Subsystem/If Action Subsystem ==
  Input : Inport
  Input1 : Inport  Port=2
  Action Port : ActionPort  ActionPortLabel=if(u1 > 0)
  Byte Unpack{,1..7} (8 alike) : etargetslib/Byte Unpack  dimensions={[1]}  datatypes={'uint16'}  byteAlign=1
      settings: SourceProductName=MATLAB Coder
  CAN Unpack : canmsglib/CAN Unpack  MsgList=(none)  MsgName=ADC A0  MsgIDType=Standard (11-bit identifier)  MsgIdentifier=CAN_ID_RAW_A0  MsgLength=2  SignalInfo=A0$0$16$1$1$1$0$1$0$-Inf$Inf$#  NSignals=1  IDPort=off  TimestampPort=off  ErrorPort=off  RemotePort=off  LengthPort=off  StatusPort=off  StartBits=str2num('[int32(0)]')  SignalSizes=str2num('[int32(16)]')  ByteOrders=str2num('[int32(1)]')  DataTypes=str2num('[int32(1)]')  MultiplexTypes=str2num('[int32(1)]')  MultiplexValues=str2num('[double(0)]')  Factors=str2num('[double(1)]')  Offsets=str2num('[double(0)]')  Minimums=str2num('[double(-Inf)]')  Maximums=str2num('[double(Inf)]')  ApplyMinMax=off
      settings: SourceProductName=Vehicle Network Toolbox  SourceProductBaseCode=VN  DataFormat=raw data
  CAN Unpack1 : canmsglib/CAN Unpack  MsgList=(none)  MsgName=ADC A1  MsgIDType=Standard (11-bit identifier)  MsgIdentifier=CAN_ID_RAW_A1  MsgLength=2  SignalInfo=A1$0$16$1$1$1$0$1$0$-Inf$Inf$#  NSignals=1  IDPort=off  TimestampPort=off  ErrorPort=off  RemotePort=off  LengthPort=off  StatusPort=off  StartBits=str2num('[int32(0)]')  SignalSizes=str2num('[int32(16)]')  ByteOrders=str2num('[int32(1)]')  DataTypes=str2num('[int32(1)]')  MultiplexTypes=str2num('[int32(1)]')  MultiplexValues=str2num('[double(0)]')  Factors=str2num('[double(1)]')  Offsets=str2num('[double(0)]')  Minimums=str2num('[double(-Inf)]')  Maximums=str2num('[double(Inf)]')  ApplyMinMax=off
      settings: SourceProductName=Vehicle Network Toolbox  SourceProductBaseCode=VN  DataFormat=raw data
  CAN Unpack2 : canmsglib/CAN Unpack  MsgList=(none)  MsgName=ADC B0  MsgIDType=Standard (11-bit identifier)  MsgIdentifier=CAN_ID_RAW_B0  MsgLength=2  SignalInfo=B0$0$16$1$1$1$0$1$0$-Inf$Inf$#  NSignals=1  IDPort=off  TimestampPort=off  ErrorPort=off  RemotePort=off  LengthPort=off  StatusPort=off  StartBits=str2num('[int32(0)]')  SignalSizes=str2num('[int32(16)]')  ByteOrders=str2num('[int32(1)]')  DataTypes=str2num('[int32(1)]')  MultiplexTypes=str2num('[int32(1)]')  MultiplexValues=str2num('[double(0)]')  Factors=str2num('[double(1)]')  Offsets=str2num('[double(0)]')  Minimums=str2num('[double(-Inf)]')  Maximums=str2num('[double(Inf)]')  ApplyMinMax=off
      settings: SourceProductName=Vehicle Network Toolbox  SourceProductBaseCode=VN  DataFormat=raw data
  CAN Unpack3 : canmsglib/CAN Unpack  MsgList=(none)  MsgName=ADC B1  MsgIDType=Standard (11-bit identifier)  MsgIdentifier=CAN_ID_RAW_B1  MsgLength=2  SignalInfo=B1$0$16$1$1$1$0$1$0$-Inf$Inf$#  NSignals=1  IDPort=off  TimestampPort=off  ErrorPort=off  RemotePort=off  LengthPort=off  StatusPort=off  StartBits=str2num('[int32(0)]')  SignalSizes=str2num('[int32(16)]')  ByteOrders=str2num('[int32(1)]')  DataTypes=str2num('[int32(1)]')  MultiplexTypes=str2num('[int32(1)]')  MultiplexValues=str2num('[double(0)]')  Factors=str2num('[double(1)]')  Offsets=str2num('[double(0)]')  Minimums=str2num('[double(-Inf)]')  Maximums=str2num('[double(Inf)]')  ApplyMinMax=off
      settings: SourceProductName=Vehicle Network Toolbox  SourceProductBaseCode=VN  DataFormat=raw data
  CAN Unpack4 : canmsglib/CAN Unpack  MsgList=(none)  MsgName=ADC C0  MsgIDType=Standard (11-bit identifier)  MsgIdentifier=CAN_ID_RAW_C0  MsgLength=2  SignalInfo=C0$0$16$1$1$1$0$1$0$-Inf$Inf$#  NSignals=1  IDPort=off  TimestampPort=off  ErrorPort=off  RemotePort=off  LengthPort=off  StatusPort=off  StartBits=str2num('[int32(0)]')  SignalSizes=str2num('[int32(16)]')  ByteOrders=str2num('[int32(1)]')  DataTypes=str2num('[int32(1)]')  MultiplexTypes=str2num('[int32(1)]')  MultiplexValues=str2num('[double(0)]')  Factors=str2num('[double(1)]')  Offsets=str2num('[double(0)]')  Minimums=str2num('[double(-Inf)]')  Maximums=str2num('[double(Inf)]')  ApplyMinMax=off
      settings: SourceProductName=Vehicle Network Toolbox  SourceProductBaseCode=VN  DataFormat=raw data
  CAN Unpack5 : canmsglib/CAN Unpack  MsgList=(none)  MsgName=ADC C1  MsgIDType=Standard (11-bit identifier)  MsgIdentifier=CAN_ID_RAW_C1  MsgLength=2  SignalInfo=C1$0$16$1$1$1$0$1$0$-Inf$Inf$#  NSignals=1  IDPort=off  TimestampPort=off  ErrorPort=off  RemotePort=off  LengthPort=off  StatusPort=off  StartBits=str2num('[int32(0)]')  SignalSizes=str2num('[int32(16)]')  ByteOrders=str2num('[int32(1)]')  DataTypes=str2num('[int32(1)]')  MultiplexTypes=str2num('[int32(1)]')  MultiplexValues=str2num('[double(0)]')  Factors=str2num('[double(1)]')  Offsets=str2num('[double(0)]')  Minimums=str2num('[double(-Inf)]')  Maximums=str2num('[double(Inf)]')  ApplyMinMax=off
      settings: SourceProductName=Vehicle Network Toolbox  SourceProductBaseCode=VN  DataFormat=raw data
  CAN Unpack6 : canmsglib/CAN Unpack  MsgList=(none)  MsgName=ADC D0  MsgIDType=Standard (11-bit identifier)  MsgIdentifier=CAN_ID_RAW_D0  MsgLength=2  SignalInfo=D0$0$16$1$1$1$0$1$0$-Inf$Inf$#  NSignals=1  IDPort=off  TimestampPort=off  ErrorPort=off  RemotePort=off  LengthPort=off  StatusPort=off  StartBits=str2num('[int32(0)]')  SignalSizes=str2num('[int32(16)]')  ByteOrders=str2num('[int32(1)]')  DataTypes=str2num('[int32(1)]')  MultiplexTypes=str2num('[int32(1)]')  MultiplexValues=str2num('[double(0)]')  Factors=str2num('[double(1)]')  Offsets=str2num('[double(0)]')  Minimums=str2num('[double(-Inf)]')  Maximums=str2num('[double(Inf)]')  ApplyMinMax=off
      settings: SourceProductName=Vehicle Network Toolbox  SourceProductBaseCode=VN  DataFormat=raw data
  CAN Unpack7 : canmsglib/CAN Unpack  MsgList=(none)  MsgName=ADC D1  MsgIDType=Standard (11-bit identifier)  MsgIdentifier=CAN_ID_RAW_D1  MsgLength=2  SignalInfo=D1$0$16$1$1$1$0$1$0$-Inf$Inf$#  NSignals=1  IDPort=off  TimestampPort=off  ErrorPort=off  RemotePort=off  LengthPort=off  StatusPort=off  StartBits=str2num('[int32(0)]')  SignalSizes=str2num('[int32(16)]')  ByteOrders=str2num('[int32(1)]')  DataTypes=str2num('[int32(1)]')  MultiplexTypes=str2num('[int32(1)]')  MultiplexValues=str2num('[double(0)]')  Factors=str2num('[double(1)]')  Offsets=str2num('[double(0)]')  Minimums=str2num('[double(-Inf)]')  Maximums=str2num('[double(Inf)]')  ApplyMinMax=off
      settings: SourceProductName=Vehicle Network Toolbox  SourceProductBaseCode=VN  DataFormat=raw data
  Constant{2..9} (8 alike) : Constant  Value=32767
  Display{3..18} (16 alike) : Display
      settings: Format=decimal (Stored Integer)
  Divide{2..9} (8 alike) : Product  Inputs=*/
  Multiply{2..9} (8 alike) : Gain  Gain=5
  Switch{2..9} (8 alike) : Switch  Criteria=u2 > Threshold
  Output2 : Outport
  Output3 : Outport  Port=2
  Output4 : Outport  Port=3
  Output5 : Outport  Port=4
  Output6 : Outport  Port=5
  Output7 : Outport  Port=6
  Output8 : Outport  Port=7
  Output9 : Outport  Port=8
  wires:
  Input1/1 -> CAN Unpack7/1, CAN Unpack6/1, CAN Unpack5/1, CAN Unpack4/1, CAN Unpack3/1, CAN Unpack2/1, CAN Unpack1/1, CAN Unpack/1  "D1"
  Switch6/1 -> Output6/1  "C1"
  CAN Unpack1/1 -> Byte Unpack1/1
  Divide7/1 -> Multiply7/1
  Byte Unpack4/1 -> Divide5/1, Switch5/3, Display12/1
  Constant5/1 -> Divide5/2
  Multiply5/1 -> Switch5/1, Display9/1
  Switch2/1 -> Output2/1  "A1"
  Divide4/1 -> Multiply4/1
  Multiply4/1 -> Switch4/1, Display7/1
  Constant4/1 -> Divide4/2
  Constant3/1 -> Divide3/2
  Byte Unpack3/1 -> Divide4/1, Switch4/3, Display8/1
  Divide3/1 -> Multiply3/1
  Switch5/1 -> Output5/1  "C0"
  Multiply8/1 -> Switch8/1, Display17/1
  Byte Unpack/1 -> Divide9/1, Switch9/3, Display11/1
  Switch8/1 -> Output8/1  "D1"
  Multiply3/1 -> Switch3/1, Display5/1
  Byte Unpack7/1 -> Divide8/1, Switch8/3, Display18/1
  Divide9/1 -> Multiply9/1
  Constant2/1 -> Divide2/2
  Switch7/1 -> Output7/1  "D0"
  Input/1 -> Switch8/2, Switch7/2, Switch6/2, Switch5/2, Switch4/2, Switch3/2, Switch2/2, Switch9/2  "int16 (0) / double (1)"
  Divide5/1 -> Multiply5/1
  Multiply6/1 -> Switch6/1, Display13/1
  Constant9/1 -> Divide9/2
  Switch9/1 -> Output9/1  "A0"
  Divide8/1 -> Multiply8/1
  Multiply2/1 -> Switch2/1, Display3/1
  Byte Unpack5/1 -> Divide6/1, Switch6/3, Display14/1
  Divide6/1 -> Multiply6/1
  Byte Unpack6/1 -> Divide7/1, Switch7/3, Display16/1
  Constant7/1 -> Divide7/2
  Multiply7/1 -> Switch7/1, Display15/1
  Byte Unpack2/1 -> Divide3/1, Switch3/3, Display6/1
  Switch3/1 -> Output3/1  "B0"
  Divide2/1 -> Multiply2/1
  Switch4/1 -> Output4/1  "B1"
  CAN Unpack5/1 -> Byte Unpack5/1
  CAN Unpack7/1 -> Byte Unpack7/1
  CAN Unpack4/1 -> Byte Unpack4/1
  Constant6/1 -> Divide6/2
  CAN Unpack3/1 -> Byte Unpack3/1
  CAN Unpack/1 -> Byte Unpack/1
  CAN Unpack6/1 -> Byte Unpack6/1
  Multiply9/1 -> Switch9/1, Display10/1
  CAN Unpack2/1 -> Byte Unpack2/1
  Constant8/1 -> Divide8/2
  Byte Unpack1/1 -> Divide2/1, Switch2/3, Display4/1

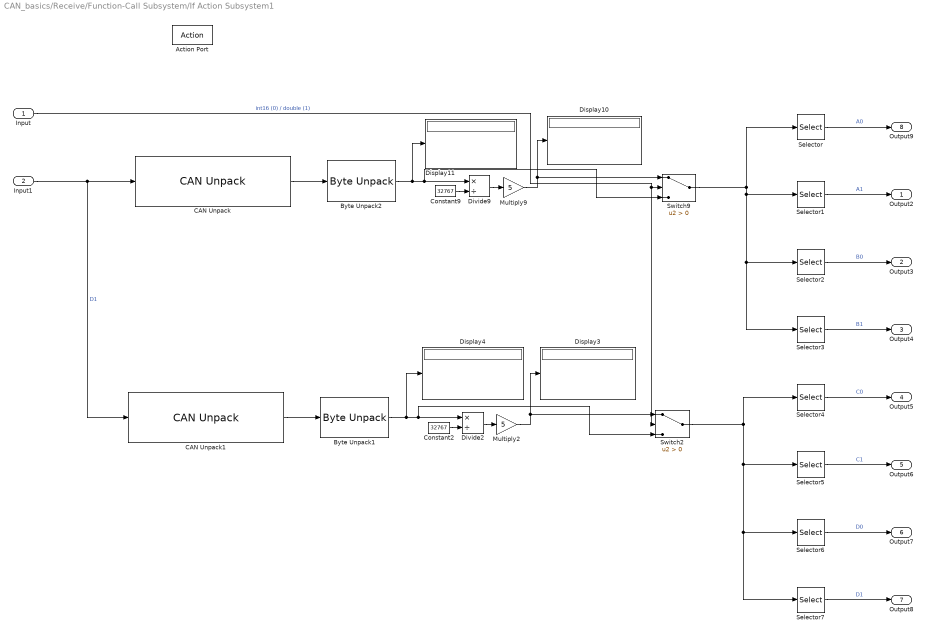
== system CAN_basics/Receive/Function-Call Subsystem/If Action Subsystem1 ==
  Input : Inport
  Input1 : Inport  Port=2
  Action Port : ActionPort  ActionPortLabel=else
  Byte Unpack1 : etargetslib/Byte Unpack  dimensions={[4]}  datatypes={'uint16'}  byteAlign=1
      settings: SourceProductName=MATLAB Coder
  Byte Unpack2 : etargetslib/Byte Unpack  dimensions={[4]}  datatypes={'uint16'}  byteAlign=1
      settings: SourceProductName=MATLAB Coder
  CAN Unpack : canmsglib/CAN Unpack  MsgList=(none)  MsgName=CAN_ID_RAW_A0  MsgIDType=Standard (11-bit identifier)  MsgIdentifier=CAN_ID_RAW_A0  MsgLength=8  SignalInfo=A0$0$16$1$1$1$0$1$0$-Inf$Inf$#  NSignals=1  IDPort=off  TimestampPort=off  ErrorPort=off  RemotePort=off  LengthPort=off  StatusPort=off  StartBits=str2num('[int32(0)]')  SignalSizes=str2num('[int32(16)]')  ByteOrders=str2num('[int32(1)]')  DataTypes=str2num('[int32(1)]')  MultiplexTypes=str2num('[int32(1)]')  MultiplexValues=str2num('[double(0)]')  Factors=str2num('[double(1)]')  Offsets=str2num('[double(0)]')  Minimums=str2num('[double(-Inf)]')  Maximums=str2num('[double(Inf)]')  ApplyMinMax=off
      settings: SourceProductName=Vehicle Network Toolbox  SourceProductBaseCode=VN  DataFormat=raw data
  CAN Unpack1 : canmsglib/CAN Unpack  MsgList=(none)  MsgName=ADC A1  MsgIDType=Standard (11-bit identifier)  MsgIdentifier=CAN_ID_RAW_A1  MsgLength=8  SignalInfo=A1$0$16$1$1$1$0$1$0$-Inf$Inf$#  NSignals=1  IDPort=off  TimestampPort=off  ErrorPort=off  RemotePort=off  LengthPort=off  StatusPort=off  StartBits=str2num('[int32(0)]')  SignalSizes=str2num('[int32(16)]')  ByteOrders=str2num('[int32(1)]')  DataTypes=str2num('[int32(1)]')  MultiplexTypes=str2num('[int32(1)]')  MultiplexValues=str2num('[double(0)]')  Factors=str2num('[double(1)]')  Offsets=str2num('[double(0)]')  Minimums=str2num('[double(-Inf)]')  Maximums=str2num('[double(Inf)]')  ApplyMinMax=off
      settings: SourceProductName=Vehicle Network Toolbox  SourceProductBaseCode=VN  DataFormat=raw data
  Constant2 : Constant  Value=32767
  Constant9 : Constant  Value=32767
  Display{3..4,10..11} (4 alike) : Display
      settings: Format=decimal (Stored Integer)
  Divide2 : Product  Inputs=*/
  Divide9 : Product  Inputs=*/
  Multiply2 : Gain  Gain=5
  Multiply9 : Gain  Gain=5
  Selector : Selector  InputPortWidth=4  IndexOptions=Index vector (dialog)  Indices=[1]  OutputSizes=1
  Selector1 : Selector  InputPortWidth=4  IndexOptions=Index vector (dialog)  Indices=[2]  OutputSizes=1
  Selector2 : Selector  InputPortWidth=4  IndexOptions=Index vector (dialog)  Indices=[3]  OutputSizes=1
  Selector3 : Selector  InputPortWidth=4  IndexOptions=Index vector (dialog)  Indices=[4]  OutputSizes=1
  Selector4 : Selector  InputPortWidth=4  IndexOptions=Index vector (dialog)  Indices=[1]  OutputSizes=1
  Selector5 : Selector  InputPortWidth=4  IndexOptions=Index vector (dialog)  Indices=[2]  OutputSizes=1
  Selector6 : Selector  InputPortWidth=4  IndexOptions=Index vector (dialog)  Indices=[3]  OutputSizes=1
  Selector7 : Selector  InputPortWidth=4  IndexOptions=Index vector (dialog)  Indices=[4]  OutputSizes=1
  Switch2 : Switch  Criteria=u2 > Threshold
  Switch9 : Switch  Criteria=u2 > Threshold
  Output2 : Outport
  Output3 : Outport  Port=2
  Output4 : Outport  Port=3
  Output5 : Outport  Port=4
  Output6 : Outport  Port=5
  Output7 : Outport  Port=6
  Output8 : Outport  Port=7
  Output9 : Outport  Port=8
  wires:
  Input1/1 -> CAN Unpack1/1, CAN Unpack/1  "D1"
  CAN Unpack1/1 -> Byte Unpack1/1
  Switch2/1 -> Selector4/1, Selector7/1, Selector6/1, Selector5/1
  Byte Unpack2/1 -> Divide9/1, Switch9/3, Display11/1
  Divide9/1 -> Multiply9/1
  Constant2/1 -> Divide2/2
  Constant9/1 -> Divide9/2
  Multiply2/1 -> Switch2/1, Display3/1
  Divide2/1 -> Multiply2/1
  CAN Unpack/1 -> Byte Unpack2/1
  Multiply9/1 -> Switch9/1, Display10/1
  Byte Unpack1/1 -> Divide2/1, Switch2/3, Display4/1
  Input/1 -> Switch2/2, Switch9/2  "int16 (0) / double (1)"
  Switch9/1 -> Selector3/1, Selector2/1, Selector1/1, Selector/1
  Selector/1 -> Output9/1  "A0"
  Selector5/1 -> Output6/1  "C1"
  Selector3/1 -> Output4/1  "B1"
  Selector7/1 -> Output8/1  "D1"
  Selector6/1 -> Output7/1  "D0"
  Selector4/1 -> Output5/1  "C0"
  Selector2/1 -> Output3/1  "B0"
  Selector1/1 -> Output2/1  "A1"

== system CAN_basics/Receive/Save_freq/Triggered Subsystem ==
  In1 : Inport
  Trigger : TriggerPort  VariantControl=Variant
  To File : ToFile  Filename=results_freq.mat  MatrixName=results_freq  SaveFormat=Timeseries
  Out1 : Outport
  wires:
  In1/1 -> To File/1, Out1/1

== system CAN_basics/Receive/Save_time/Triggered Subsystem ==
  In1 : Inport
  Trigger : TriggerPort  VariantControl=Variant
  To File : ToFile  Filename=results_time.mat  MatrixName=results_time
  Out1 : Outport
  wires:
  In1/1 -> To File/1, Out1/1
